simulink model "sm_car_testrig_susp_dwa_hp"  (R2025b)
settings: Solver=ode23t  StartTime=0.0  StopTime=1e-9  RelTol=1e-3  EnableMultiTasking=on
PostLoadFcn:
  | sm_car_load_vehicle_data(bdroot,'016');
undefined symbols (not defined in the file): Init, LAf, LAr, UAf, UAr, Vehicle, X, Y, Z
libraries: sm_lib x102, nesl_utility x67, Suspension_Utilities x8, Linkage_Arms x6, Linkage_DW_A x4, fl_lib x4, Linkage_Shock x2, Linkage_Uprights x2
(part 3 of 4)

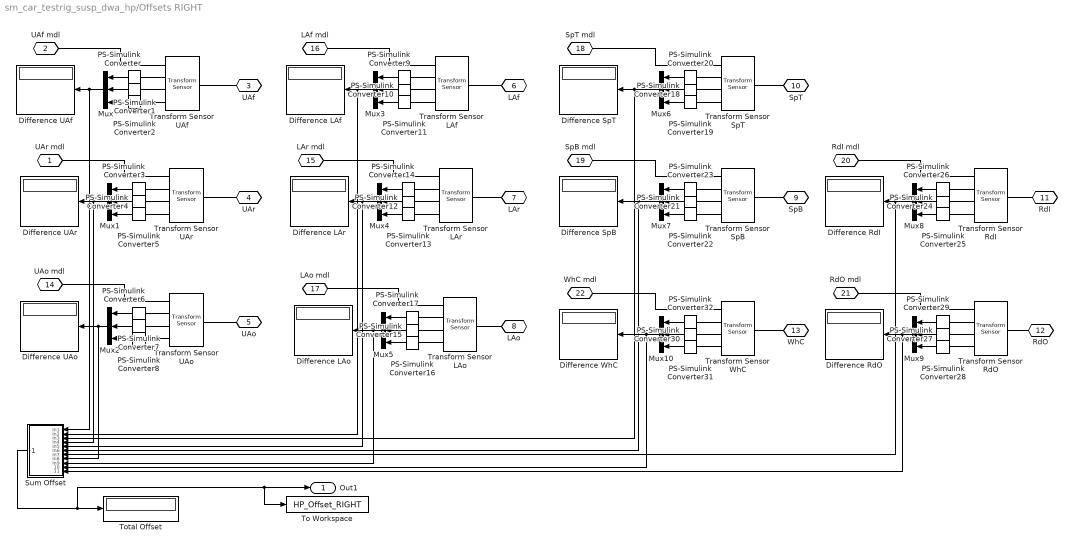
== system sm_car_testrig_susp_dwa_hp/Offsets RIGHT ==
  Difference LAf : Display
  Difference LAo : Display
  Difference LAr : Display
  Difference RdI : Display
  Difference RdO : Display
  Difference SpB : Display
  Difference SpT : Display
  Difference UAf : Display
  Difference UAo : Display
  Difference UAr : Display
  Difference WhC : Display
  Mux{,1..10} (11 alike) : Mux  Inputs=3
  PS-Simulink Converter{,1..32} (33 alike) : nesl_utility/PS-Simulink Converter  PhysicalDomain=network_engine_domain  SubClassName=ps_output  LeftPortType=input  RightPortType=output  PseudoPeriodic=off  Frequencies=[]  VectorFormat=1-D array  Unit=1  AffineConversion=off
  Sum Offset : Subsystem
  To Workspace : ToWorkspace  VariableName=HP_Offset_RIGHT  SaveFormat=Timeseries  SampleTime=-1
  Total Offset : Display
  Transform Sensor LAf : sm_lib/Frames and Transforms/Transform Sensor  MeasurementFrame=World  RotationSequence=XYX  SenseAngle=off  SenseAxis=off  SenseQ=off  SenseR=off  SenseRotationSequence=off  SenseOmegaX=off  SenseOmegaY=off  SenseOmegaZ=off  SenseOmega=off  SenseQDot=off  SenseRDot=off  SenseRotationSequenceDot=off  SenseAlphaX=off  SenseAlphaY=off  SenseAlphaZ=off  SenseAlpha=off  SenseQDDot=off  SenseRDDot=off  SenseX=on  SenseY=on  SenseZ=on  SenseXYZ=off  SenseRad=off  SenseAzim=off  SenseDist=off  SenseInc=off  SenseXDot=off  SenseYDot=off  SenseZDot=off  SenseXYZDot=off  SenseRadDot=off  SenseAzimDot=off  SenseDistDot=off  SenseIncDot=off  SenseXDDot=off  SenseYDDot=off  SenseZDDot=off  SenseXYZDDot=off  SenseRadDDot=off  SenseAzimDDot=off  SenseDistDDot=off  SenseIncDDot=off
  Transform Sensor LAo : sm_lib/Frames and Transforms/Transform Sensor  MeasurementFrame=World  RotationSequence=XYX  SenseAngle=off  SenseAxis=off  SenseQ=off  SenseR=off  SenseRotationSequence=off  SenseOmegaX=off  SenseOmegaY=off  SenseOmegaZ=off  SenseOmega=off  SenseQDot=off  SenseRDot=off  SenseRotationSequenceDot=off  SenseAlphaX=off  SenseAlphaY=off  SenseAlphaZ=off  SenseAlpha=off  SenseQDDot=off  SenseRDDot=off  SenseX=on  SenseY=on  SenseZ=on  SenseXYZ=off  SenseRad=off  SenseAzim=off  SenseDist=off  SenseInc=off  SenseXDot=off  SenseYDot=off  SenseZDot=off  SenseXYZDot=off  SenseRadDot=off  SenseAzimDot=off  SenseDistDot=off  SenseIncDot=off  SenseXDDot=off  SenseYDDot=off  SenseZDDot=off  SenseXYZDDot=off  SenseRadDDot=off  SenseAzimDDot=off  SenseDistDDot=off  SenseIncDDot=off
  Transform Sensor LAr : sm_lib/Frames and Transforms/Transform Sensor  MeasurementFrame=World  RotationSequence=XYX  SenseAngle=off  SenseAxis=off  SenseQ=off  SenseR=off  SenseRotationSequence=off  SenseOmegaX=off  SenseOmegaY=off  SenseOmegaZ=off  SenseOmega=off  SenseQDot=off  SenseRDot=off  SenseRotationSequenceDot=off  SenseAlphaX=off  SenseAlphaY=off  SenseAlphaZ=off  SenseAlpha=off  SenseQDDot=off  SenseRDDot=off  SenseX=on  SenseY=on  SenseZ=on  SenseXYZ=off  SenseRad=off  SenseAzim=off  SenseDist=off  SenseInc=off  SenseXDot=off  SenseYDot=off  SenseZDot=off  SenseXYZDot=off  SenseRadDot=off  SenseAzimDot=off  SenseDistDot=off  SenseIncDot=off  SenseXDDot=off  SenseYDDot=off  SenseZDDot=off  SenseXYZDDot=off  SenseRadDDot=off  SenseAzimDDot=off  SenseDistDDot=off  SenseIncDDot=off
  Transform Sensor RdI : sm_lib/Frames and Transforms/Transform Sensor  MeasurementFrame=World  RotationSequence=XYX  SenseAngle=off  SenseAxis=off  SenseQ=off  SenseR=off  SenseRotationSequence=off  SenseOmegaX=off  SenseOmegaY=off  SenseOmegaZ=off  SenseOmega=off  SenseQDot=off  SenseRDot=off  SenseRotationSequenceDot=off  SenseAlphaX=off  SenseAlphaY=off  SenseAlphaZ=off  SenseAlpha=off  SenseQDDot=off  SenseRDDot=off  SenseX=on  SenseY=on  SenseZ=on  SenseXYZ=off  SenseRad=off  SenseAzim=off  SenseDist=off  SenseInc=off  SenseXDot=off  SenseYDot=off  SenseZDot=off  SenseXYZDot=off  SenseRadDot=off  SenseAzimDot=off  SenseDistDot=off  SenseIncDot=off  SenseXDDot=off  SenseYDDot=off  SenseZDDot=off  SenseXYZDDot=off  SenseRadDDot=off  SenseAzimDDot=off  SenseDistDDot=off  SenseIncDDot=off
  Transform Sensor RdO : sm_lib/Frames and Transforms/Transform Sensor  MeasurementFrame=World  RotationSequence=XYX  SenseAngle=off  SenseAxis=off  SenseQ=off  SenseR=off  SenseRotationSequence=off  SenseOmegaX=off  SenseOmegaY=off  SenseOmegaZ=off  SenseOmega=off  SenseQDot=off  SenseRDot=off  SenseRotationSequenceDot=off  SenseAlphaX=off  SenseAlphaY=off  SenseAlphaZ=off  SenseAlpha=off  SenseQDDot=off  SenseRDDot=off  SenseX=on  SenseY=on  SenseZ=on  SenseXYZ=off  SenseRad=off  SenseAzim=off  SenseDist=off  SenseInc=off  SenseXDot=off  SenseYDot=off  SenseZDot=off  SenseXYZDot=off  SenseRadDot=off  SenseAzimDot=off  SenseDistDot=off  SenseIncDot=off  SenseXDDot=off  SenseYDDot=off  SenseZDDot=off  SenseXYZDDot=off  SenseRadDDot=off  SenseAzimDDot=off  SenseDistDDot=off  SenseIncDDot=off
  Transform Sensor SpB : sm_lib/Frames and Transforms/Transform Sensor  MeasurementFrame=World  RotationSequence=XYX  SenseAngle=off  SenseAxis=off  SenseQ=off  SenseR=off  SenseRotationSequence=off  SenseOmegaX=off  SenseOmegaY=off  SenseOmegaZ=off  SenseOmega=off  SenseQDot=off  SenseRDot=off  SenseRotationSequenceDot=off  SenseAlphaX=off  SenseAlphaY=off  SenseAlphaZ=off  SenseAlpha=off  SenseQDDot=off  SenseRDDot=off  SenseX=on  SenseY=on  SenseZ=on  SenseXYZ=off  SenseRad=off  SenseAzim=off  SenseDist=off  SenseInc=off  SenseXDot=off  SenseYDot=off  SenseZDot=off  SenseXYZDot=off  SenseRadDot=off  SenseAzimDot=off  SenseDistDot=off  SenseIncDot=off  SenseXDDot=off  SenseYDDot=off  SenseZDDot=off  SenseXYZDDot=off  SenseRadDDot=off  SenseAzimDDot=off  SenseDistDDot=off  SenseIncDDot=off
  Transform Sensor SpT : sm_lib/Frames and Transforms/Transform Sensor  MeasurementFrame=World  RotationSequence=XYX  SenseAngle=off  SenseAxis=off  SenseQ=off  SenseR=off  SenseRotationSequence=off  SenseOmegaX=off  SenseOmegaY=off  SenseOmegaZ=off  SenseOmega=off  SenseQDot=off  SenseRDot=off  SenseRotationSequenceDot=off  SenseAlphaX=off  SenseAlphaY=off  SenseAlphaZ=off  SenseAlpha=off  SenseQDDot=off  SenseRDDot=off  SenseX=on  SenseY=on  SenseZ=on  SenseXYZ=off  SenseRad=off  SenseAzim=off  SenseDist=off  SenseInc=off  SenseXDot=off  SenseYDot=off  SenseZDot=off  SenseXYZDot=off  SenseRadDot=off  SenseAzimDot=off  SenseDistDot=off  SenseIncDot=off  SenseXDDot=off  SenseYDDot=off  SenseZDDot=off  SenseXYZDDot=off  SenseRadDDot=off  SenseAzimDDot=off  SenseDistDDot=off  SenseIncDDot=off
  Transform Sensor UAf : sm_lib/Frames and Transforms/Transform Sensor  MeasurementFrame=World  RotationSequence=XYX  SenseAngle=off  SenseAxis=off  SenseQ=off  SenseR=off  SenseRotationSequence=off  SenseOmegaX=off  SenseOmegaY=off  SenseOmegaZ=off  SenseOmega=off  SenseQDot=off  SenseRDot=off  SenseRotationSequenceDot=off  SenseAlphaX=off  SenseAlphaY=off  SenseAlphaZ=off  SenseAlpha=off  SenseQDDot=off  SenseRDDot=off  SenseX=on  SenseY=on  SenseZ=on  SenseXYZ=off  SenseRad=off  SenseAzim=off  SenseDist=off  SenseInc=off  SenseXDot=off  SenseYDot=off  SenseZDot=off  SenseXYZDot=off  SenseRadDot=off  SenseAzimDot=off  SenseDistDot=off  SenseIncDot=off  SenseXDDot=off  SenseYDDot=off  SenseZDDot=off  SenseXYZDDot=off  SenseRadDDot=off  SenseAzimDDot=off  SenseDistDDot=off  SenseIncDDot=off
  Transform Sensor UAo : sm_lib/Frames and Transforms/Transform Sensor  MeasurementFrame=World  RotationSequence=XYX  SenseAngle=off  SenseAxis=off  SenseQ=off  SenseR=off  SenseRotationSequence=off  SenseOmegaX=off  SenseOmegaY=off  SenseOmegaZ=off  SenseOmega=off  SenseQDot=off  SenseRDot=off  SenseRotationSequenceDot=off  SenseAlphaX=off  SenseAlphaY=off  SenseAlphaZ=off  SenseAlpha=off  SenseQDDot=off  SenseRDDot=off  SenseX=on  SenseY=on  SenseZ=on  SenseXYZ=off  SenseRad=off  SenseAzim=off  SenseDist=off  SenseInc=off  SenseXDot=off  SenseYDot=off  SenseZDot=off  SenseXYZDot=off  SenseRadDot=off  SenseAzimDot=off  SenseDistDot=off  SenseIncDot=off  SenseXDDot=off  SenseYDDot=off  SenseZDDot=off  SenseXYZDDot=off  SenseRadDDot=off  SenseAzimDDot=off  SenseDistDDot=off  SenseIncDDot=off
  Transform Sensor UAr : sm_lib/Frames and Transforms/Transform Sensor  MeasurementFrame=World  RotationSequence=XYX  SenseAngle=off  SenseAxis=off  SenseQ=off  SenseR=off  SenseRotationSequence=off  SenseOmegaX=off  SenseOmegaY=off  SenseOmegaZ=off  SenseOmega=off  SenseQDot=off  SenseRDot=off  SenseRotationSequenceDot=off  SenseAlphaX=off  SenseAlphaY=off  SenseAlphaZ=off  SenseAlpha=off  SenseQDDot=off  SenseRDDot=off  SenseX=on  SenseY=on  SenseZ=on  SenseXYZ=off  SenseRad=off  SenseAzim=off  SenseDist=off  SenseInc=off  SenseXDot=off  SenseYDot=off  SenseZDot=off  SenseXYZDot=off  SenseRadDot=off  SenseAzimDot=off  SenseDistDot=off  SenseIncDot=off  SenseXDDot=off  SenseYDDot=off  SenseZDDot=off  SenseXYZDDot=off  SenseRadDDot=off  SenseAzimDDot=off  SenseDistDDot=off  SenseIncDDot=off
  Transform Sensor WhC : sm_lib/Frames and Transforms/Transform Sensor  MeasurementFrame=World  RotationSequence=XYX  SenseAngle=off  SenseAxis=off  SenseQ=off  SenseR=off  SenseRotationSequence=off  SenseOmegaX=off  SenseOmegaY=off  SenseOmegaZ=off  SenseOmega=off  SenseQDot=off  SenseRDot=off  SenseRotationSequenceDot=off  SenseAlphaX=off  SenseAlphaY=off  SenseAlphaZ=off  SenseAlpha=off  SenseQDDot=off  SenseRDDot=off  SenseX=on  SenseY=on  SenseZ=on  SenseXYZ=off  SenseRad=off  SenseAzim=off  SenseDist=off  SenseInc=off  SenseXDot=off  SenseYDot=off  SenseZDot=off  SenseXYZDot=off  SenseRadDot=off  SenseAzimDot=off  SenseDistDot=off  SenseIncDot=off  SenseXDDot=off  SenseYDDot=off  SenseZDDot=off  SenseXYZDDot=off  SenseRadDDot=off  SenseAzimDDot=off  SenseDistDDot=off  SenseIncDDot=off
  UAr mdl : PMIOPort  Side=Right
  UAf mdl : PMIOPort  Port=2  Side=Right
  UAf : PMIOPort  Port=3  Side=Left
  UAr : PMIOPort  Port=4  Side=Left
  UAo : PMIOPort  Port=5  Side=Left
  LAf : PMIOPort  Port=6  Side=Left
  LAr : PMIOPort  Port=7  Side=Left
  LAo : PMIOPort  Port=8  Side=Left
  SpB : PMIOPort  Port=9  Side=Left
  SpT : PMIOPort  Port=10  Side=Left
  RdI : PMIOPort  Port=11  Side=Left
  RdO : PMIOPort  Port=12  Side=Left
  WhC : PMIOPort  Port=13  Side=Left
  UAo mdl : PMIOPort  Port=14  Side=Right
  LAr mdl : PMIOPort  Port=15  Side=Right
  LAf mdl : PMIOPort  Port=16  Side=Right
  LAo mdl : PMIOPort  Port=17  Side=Right
  SpT mdl : PMIOPort  Port=18  Side=Right
  SpB mdl : PMIOPort  Port=19  Side=Right
  RdI mdl : PMIOPort  Port=20  Side=Right
  RdO mdl : PMIOPort  Port=21  Side=Right
  WhC mdl : PMIOPort  Port=22  Side=Right
  Out1 : Outport  VectorParamsAs1DForOutWhenUnconnected=off
  wires:
  Sum Offset/1(Out1) -> To Workspace/1, Out1/1, Total Offset/1
  PS-Simulink Converter32/1 -> Mux10/1
  PS-Simulink Converter31/1 -> Mux10/3
  PS-Simulink Converter30/1 -> Mux10/2
  Mux10/1 -> Difference WhC/1, Sum Offset/10(In10)
  Mux9/1 -> Difference RdO/1, Sum Offset/11(In11)
  PS-Simulink Converter27/1 -> Mux9/2
  PS-Simulink Converter28/1 -> Mux9/3
  PS-Simulink Converter29/1 -> Mux9/1
  PS-Simulink Converter26/1 -> Mux8/1
  PS-Simulink Converter25/1 -> Mux8/3
  PS-Simulink Converter24/1 -> Mux8/2
  Mux8/1 -> Difference RdI/1, Sum Offset/7(In7)
  Mux7/1 -> Difference SpB/1, Sum Offset/6(In6)
  PS-Simulink Converter21/1 -> Mux7/2
  PS-Simulink Converter22/1 -> Mux7/3
  PS-Simulink Converter23/1 -> Mux7/1
  PS-Simulink Converter20/1 -> Mux6/1
  PS-Simulink Converter19/1 -> Mux6/3
  PS-Simulink Converter18/1 -> Mux6/2
  Mux6/1 -> Difference SpT/1, Sum Offset/3(In3)
  Mux5/1 -> Difference LAo/1, Sum Offset/9(In9)
  PS-Simulink Converter15/1 -> Mux5/2
  PS-Simulink Converter16/1 -> Mux5/3
  PS-Simulink Converter17/1 -> Mux5/1
  PS-Simulink Converter14/1 -> Mux4/1
  PS-Simulink Converter13/1 -> Mux4/3
  PS-Simulink Converter12/1 -> Mux4/2
  Mux4/1 -> Difference LAr/1, Sum Offset/5(In5)
  Mux3/1 -> Difference LAf/1, Sum Offset/2(In2)
  PS-Simulink Converter10/1 -> Mux3/2
  PS-Simulink Converter11/1 -> Mux3/3
  PS-Simulink Converter9/1 -> Mux3/1
  PS-Simulink Converter6/1 -> Mux2/1
  PS-Simulink Converter8/1 -> Mux2/3
  PS-Simulink Converter7/1 -> Mux2/2
  Mux2/1 -> Difference UAo/1, Sum Offset/8(In8)
  Mux1/1 -> Difference UAr/1, Sum Offset/4(In4)
  PS-Simulink Converter4/1 -> Mux1/2
  PS-Simulink Converter5/1 -> Mux1/3
  PS-Simulink Converter3/1 -> Mux1/1
  PS-Simulink Converter/1 -> Mux/1
  PS-Simulink Converter2/1 -> Mux/3
  PS-Simulink Converter1/1 -> Mux/2
  Mux/1 -> Difference UAf/1, Sum Offset/1(In1)
  connections:
  WhC/RConn1 -- Transform Sensor WhC/LConn1
  Transform Sensor WhC/RConn1 -- WhC mdl/RConn1
  Transform Sensor WhC/RConn2 -- PS-Simulink Converter32/LConn1
  PS-Simulink Converter30/LConn1 -- Transform Sensor WhC/RConn3
  PS-Simulink Converter31/LConn1 -- Transform Sensor WhC/RConn4
  Transform Sensor RdO/RConn1 -- RdO mdl/RConn1
  PS-Simulink Converter28/LConn1 -- Transform Sensor RdO/RConn4
  PS-Simulink Converter27/LConn1 -- Transform Sensor RdO/RConn3
  Transform Sensor RdO/RConn2 -- PS-Simulink Converter29/LConn1
  RdO/RConn1 -- Transform Sensor RdO/LConn1
  RdI/RConn1 -- Transform Sensor RdI/LConn1
  Transform Sensor RdI/RConn1 -- RdI mdl/RConn1
  Transform Sensor RdI/RConn2 -- PS-Simulink Converter26/LConn1
  PS-Simulink Converter24/LConn1 -- Transform Sensor RdI/RConn3
  PS-Simulink Converter25/LConn1 -- Transform Sensor RdI/RConn4
  PS-Simulink Converter22/LConn1 -- Transform Sensor SpB/RConn4
  PS-Simulink Converter21/LConn1 -- Transform Sensor SpB/RConn3
  Transform Sensor SpB/RConn1 -- SpB mdl/RConn1
  Transform Sensor SpB/RConn2 -- PS-Simulink Converter23/LConn1
  SpB/RConn1 -- Transform Sensor SpB/LConn1
  SpT/RConn1 -- Transform Sensor SpT/LConn1
  Transform Sensor SpT/RConn1 -- SpT mdl/RConn1
  Transform Sensor SpT/RConn2 -- PS-Simulink Converter20/LConn1
  PS-Simulink Converter18/LConn1 -- Transform Sensor SpT/RConn3
  PS-Simulink Converter19/LConn1 -- Transform Sensor SpT/RConn4
  Transform Sensor LAo/RConn1 -- LAo mdl/RConn1
  Transform Sensor LAo/RConn2 -- PS-Simulink Converter17/LConn1
  PS-Simulink Converter16/LConn1 -- Transform Sensor LAo/RConn4
  PS-Simulink Converter15/LConn1 -- Transform Sensor LAo/RConn3
  LAo/RConn1 -- Transform Sensor LAo/LConn1
  LAr/RConn1 -- Transform Sensor LAr/LConn1
  Transform Sensor LAr/RConn1 -- LAr mdl/RConn1
  Transform Sensor LAr/RConn2 -- PS-Simulink Converter14/LConn1
  PS-Simulink Converter12/LConn1 -- Transform Sensor LAr/RConn3
  PS-Simulink Converter13/LConn1 -- Transform Sensor LAr/RConn4
  PS-Simulink Converter11/LConn1 -- Transform Sensor LAf/RConn4
  PS-Simulink Converter10/LConn1 -- Transform Sensor LAf/RConn3
  LAf/RConn1 -- Transform Sensor LAf/LConn1
  Transform Sensor LAf/RConn2 -- PS-Simulink Converter9/LConn1
  Transform Sensor LAf/RConn1 -- LAf mdl/RConn1
  Transform Sensor UAo/RConn2 -- PS-Simulink Converter6/LConn1
  UAo mdl/RConn1 -- Transform Sensor UAo/RConn1
  PS-Simulink Converter8/LConn1 -- Transform Sensor UAo/RConn4
  UAo/RConn1 -- Transform Sensor UAo/LConn1
  PS-Simulink Converter7/LConn1 -- Transform Sensor UAo/RConn3
  PS-Simulink Converter5/LConn1 -- Transform Sensor UAr/RConn4
  PS-Simulink Converter4/LConn1 -- Transform Sensor UAr/RConn3
  UAr/RConn1 -- Transform Sensor UAr/LConn1
  Transform Sensor UAr/RConn2 -- PS-Simulink Converter3/LConn1
  UAr mdl/RConn1 -- Transform Sensor UAr/RConn1
  Transform Sensor UAf/RConn1 -- UAf mdl/RConn1
  Transform Sensor UAf/RConn2 -- PS-Simulink Converter/LConn1
  Transform Sensor UAf/LConn1 -- UAf/RConn1
  PS-Simulink Converter1/LConn1 -- Transform Sensor UAf/RConn3
  PS-Simulink Converter2/LConn1 -- Transform Sensor UAf/RConn4
